simulink model "Observadores_Mimo"  (R2022b)
settings: Solver=ode23t  StartTime=0.0  StopTime=5  MaxStep=1e-3  RelTol=1e-3
values from neighbouring files (symbols this model uses):
  Ac = reg.a    [Observdores_funcion_lqg.m]    (also in Observdores_pto_equilibrio.m)
  Ac_1 = [AL-BL*Kest-L*CL+L*DL*Kest, BL*Ki - L*DL*Ki ... (first row only)    [Observdores.m]
  Ac_2 = reg.a    [Observdores.m]    (also in Observdores_funcion_lqg.m; lqg_funcion.m)
  AL = double(subs(A,{a,b,c,d},{a1,b1,c1,d1}))    [Observdores.m]    (also in Observdores_funcion_lqg.m = double(subs(A,{x1,x2,x3,x4,u1,u2,u3,u4},{x10,x20,x30,x40,u10; Observdores_pto_equilibrio.m; Observdores_pto_equilibrio_discreto.m; Observdores_seguimiento_discreto.m)
  Bc = reg.b    [Observdores_funcion_lqg.m]    (also in Observdores_pto_equilibrio.m)
  Bc_1 = [-L ... (first row only)    [Observdores.m]
  Bc_2 = reg.b    [Observdores.m]    (also in Observdores_funcion_lqg.m; lqg_funcion.m)
  BL = double(subs(B,{a,b,c,d},{a1,b1,c1,d1}))    [Observdores.m]    (also in Observdores_funcion_lqg.m = double(subs(B,{x1,x2,x3,x4,u1,u2,u3,u4},{x10,x20,x30,x40,u10; Observdores_pto_equilibrio.m; Observdores_pto_equilibrio_discreto.m; Observdores_seguimiento_discreto.m)
  Cc = sys_d2.c    [Observdores.m]    (also in Observdores_funcion_lqg.m = reg.c; Observdores_pto_equilibrio.m = reg.c; Observdores_pto_equilibrio_discreto.m = -K)
  Cc_1 = [-Kest, Ki]    [Observdores.m]
  Cc_2 = reg.c    [Observdores.m]    (also in Observdores_funcion_lqg.m; lqg_funcion.m)
  Ccon = [-Kest Ki]    [Observdores_seguimiento_discreto.m]
  CL = [1 0 0 ... (first row only)    [Observdores.m]    (also in Observdores_funcion_lqg.m = [1 1 0 0; Observdores_pto_equilibrio.m; Observdores_pto_equilibrio_discreto.m; Observdores_seguimiento_discreto.m)
  Dc = reg.d    [Observdores_funcion_lqg.m]    (also in Observdores_pto_equilibrio.m; Observdores_pto_equilibrio_discreto.m = zeros(p,r))
  Dc_1 = zeros(p,r)    [Observdores.m]
  Dc_2 = reg.d    [Observdores.m]    (also in Observdores_funcion_lqg.m; lqg_funcion.m)
  Dcon = zeros(p,2*r)    [Observdores_seguimiento_discreto.m]
  DL = [0 0 0 ... (first row only)    [Observdores.m]    (also in Observdores_funcion_lqg.m = [0 0 0 0; Observdores_pto_equilibrio.m; Observdores_pto_equilibrio_discreto.m; Observdores_seguimiento_discreto.m)
  Gc = sys_d2.a    [Observdores.m]    (also in Observdores_pto_equilibrio.m = sys_c_dig.a; Observdores_pto_equilibrio_discreto.m = GL-HL*K-L*CL+L*DL*K)
  Gcon = [GL-HL*Kest-L*CL+L*DL*Kest, HL*Ki - L*DL*Ki ... (first row only)    [Observdores_seguimiento_discreto.m]
  GL = sysd.a    [Observdores_pto_equilibrio_discreto.m]    (also in Observdores_seguimiento_discreto.m)
  Hc = sys_c_dig.b    [Observdores_pto_equilibrio.m]    (also in Observdores_pto_equilibrio_discreto.m = L)
  Hcon = [zeros(n,r), L ... (first row only)    [Observdores_seguimiento_discreto.m]
  HL = sysd.b    [Observdores_pto_equilibrio_discreto.m]    (also in Observdores_seguimiento_discreto.m)
  K = place(Ahat,Bhat,delta)    [Observdores.m]
  Kest = K(:,1:n)    [Observdores.m]    (also in Observdores_seguimiento_discreto.m)
  Ki = -K(:,n+1:end)    [Observdores.m]    (also in Observdores_seguimiento_discreto.m)
  L = (place(AL',CL',delta))'    [Observdores.m]    (also in Observdores_pto_equilibrio.m; Observdores_pto_equilibrio_discreto.m = place(GL',CL',pol_obv_d)'; Observdores_seguimiento_discreto.m = place(GL',CL',pol_obv_d)')
  sys_d1 = c2d(sys_c1,Tm)    [Observdores.m]
  sys_d2 = c2d(sys_c2,Tm)    [Observdores.m]
  Tm = 0.02    [Observdores.m]    (also in Observdores_pto_equilibrio.m; Observdores_pto_equilibrio_discreto.m = 0.05; Observdores_seguimiento_discreto.m = 0.05)
  u10 = (a1*x20 + b1*x10^2)/u20    [Observdores.m]    (also in Observdores_funcion_lqg.m = 1; Observdores_pto_equilibrio.m; Observdores_pto_equilibrio_discreto.m; Observdores_seguimiento_discreto.m)
  u20 = sqrt(c1*x30*x20)    [Observdores.m]    (also in Observdores_funcion_lqg.m = sqrt(x30*x20); Observdores_pto_equilibrio.m; Observdores_pto_equilibrio_discreto.m; Observdores_seguimiento_discreto.m)
  u30 = (d1*x30 - u10)/x10    [Observdores.m]    (also in Observdores_funcion_lqg.m = (x20 + x10^2 - u20^2)/u10; Observdores_pto_equilibrio.m; Observdores_pto_equilibrio_discreto.m; Observdores_seguimiento_discreto.m)
  x10 = 2    [Observdores.m]    (also in Observdores_funcion_lqg.m; Observdores_pto_equilibrio.m; Observdores_pto_equilibrio_discreto.m; Observdores_seguimiento_discreto.m)
  x20 = 4    [Observdores.m]    (also in Observdores_funcion_lqg.m = 8; Observdores_pto_equilibrio.m; Observdores_pto_equilibrio_discreto.m; Observdores_seguimiento_discreto.m)
  x30 = 4    [Observdores.m]    (also in Observdores_funcion_lqg.m = 2; Observdores_pto_equilibrio.m; Observdores_pto_equilibrio_discreto.m; Observdores_seguimiento_discreto.m)
  xini = [0.5; -0.3; -0.7; 0.9]    [Observdores_funcion_lqg.m]    (also in Observdores_pto_equilibrio.m = [0.2; -0.3; -0.4]; Observdores_pto_equilibrio_discreto.m = [0.2; -0.3; -0.4])
undefined symbols (not defined in the file or in its folder): magnitude
libraries: simulink x22
(part 3 of 3)

== matlab function Observadores_Mimo/Comparacion/MATLAB Function3 ==
  data: Sp input; ut output; Pv input; Con_in input; Con_out output
function [ut,Con_out] = fcn(Sp,Pv,Con_in)
Vk_1 = Con_in(1:2); % Número de integradores
Xk_1 = Con_in(3:5); % Estados planta
Du = Con_in(6:8); % Actuadores

u1max = 10;
u1min = -10;
u2max = 10;
u2min = -10;
u3max = 10;
u3min = -10;
u4max = 10;
u4min = -10;
Ka = zeros(2,3);  %(r,p)

GL = [0.449639072151396	-0.0615751578519137	0.00688879884775241
-0.0103331982716286	0.819090019262878	-0.167927508214218
0.0949460363457777	-0.00516659913581431	0.861071896316432];
HL = [0.137811004816424	0.191992740153676	0.000252311833454837
-0.00521058225806007	0.361441493724063	-0.00890729351539111
0.0575256575832432	0.0158782651576252	0.0928710476225001];
CL = [1	0	0
0	0	1];
Ki = [0.495926463268089	0.0790916425769034
0.300095646296171	0.0155567242100712
-0.211852960593149	0.275825414863402];
Kest = [0.507477329350552	-0.352045881677806	0.562420881396554
0.247771497752502	0.347060818569204	-0.103614364293038
0.0518961155196881	0.0183168185614278	1.23984083631819];
L = [0.0236567937142856	0.00882380149521764
0.0520705602169565	-0.0103631100189368
0.0214783272972567	0.0442958071558840];

en = Sp-Pv;
Vk = en + Vk_1 - Ka*Du;
u = Ki*Vk - Kest*Xk_1;
Xob = (GL-L*CL)*Xk_1 + HL*u + L*Pv;

u1s = u(1);
u2s = u(2);
u3s = u(3);

if u(1)>=u1max
    u1s = u1max;
end
if u(1)<=u1min
    u1s = u1min;
end

if u(2)>=u2max
    u2s = u2max;
end
if u(2)<=u2min
    u2s = u2min;
end

if u(3)>=u3max
    u3s = u3max;
end
if u(3)<=u3min
    u3s = u3min;
end

%% Salida
ut = [u1s;u2s;u3s];
Dunew = u - ut;
Con_out = [Vk; Xob; Dunew];

== matlab function Observadores_Mimo/Comparacion/Subsystem6/MATLAB Function ==
  data: x input; f output; u1 input; u2 input; u3 input
function f = fcn(x,u1,u2,u3)

x1 = x(1);
x2 = x(2);
x3 = x(3);

a = 2;
b = 4;
c = 1;
d = 3;

f1 = -a*x2 - b*x1^2 + u1*u2;
f2 = -c*x3*x2 + u2^2 ;
f3 = -d*x3 + u3*x1 + u1;

f = [f1;f2;f3];

== matlab function Observadores_Mimo/Control Estados_1 DOF_Unificado/MATLAB Function2 ==
  data: Sp input; ut output; Pv input; Con_ini input; Con_out output
function [ut,Con_out] = fcn(Sp,Pv,Con_ini)
Gc = [0.939974592711359	-2.37159326323049e-12	-0.00286835310590601	0.0698167323415246	-0.00133465785652806
-0.000328954995677950	0.802518797962479	0.00531052595531562	-1.22918191880968e-05	0.00254152882572689
-0.00286835310583805	4.00834161597228e-15	0.759858388826903	-0.000109199276806931	0.769506721453615
0	0	0	1	0
0	0	0	0	1];
Hc = [-0.00537081940417820	-0.00326725714133668
-0.000338557035146039	0.00607025843071000
-0.00295366005744958	-0.00876393614924446
0.0100000000000000	0
0	0.0100000000000000];
Cc = [2.60000000006463	3.87499999993181	-0.750000000024670	1.79999999984347	9.96447369061571e-11
-4.30872282297656e-11	-2.25000000000000	0.499999999999999	1.04354552776798e-10	1.64313007644523e-14
-2.80000000007810	-1.93749999996589	-11.1249999999877	-0.899999999768644	43.9999999999502];
Dc = [0	0
0	0
0	0];

u1max = 10;
u1min = -10;
u2max = 10;
u2min = -10;
u3max = 10;
u3min = -10;

Ka = zeros(5,3);  % (n+r,p)

xk = Con_ini(1:5);  %n+r
Du = Con_ini(6:8);  %p

error = Sp-Pv;
u = Cc*xk + Dc*error;
xk_1 = Gc*xk + Hc*error - Ka*Du;

u1s = u(1);
u2s = u(2);
u3s = u(3);

if u(1)>=u1max
    u1s = u1max;
end
if u(1)<=u1min
    u1s = u1min;
end

if u(2)>=u2max
    u2s = u2max;
end
if u(2)<=u2min
    u2s = u2min;
end

if u(3)>=u3max
    u3s = u3max;
end
if u(3)<=u3min
    u3s = u3min;
end

%% Salida
ut = [u1s;u2s;u3s];
Dunew = u - ut;
Con_out = [xk_1; Dunew];

== matlab function Observadores_Mimo/Control Estados_Punto Equilibrio_Discret_Codigo/MATLAB Function ==
  data: Pv input; ut output; Con_ini input; Con_out output
function [ut,Con_out] = fcn(Pv,Con_ini)
Gc = [0.423094793522468	-0.0746380079945671	7.31048780287791e-06
-0.0636860426356503	0.790816757730642	-0.142538588641518
0.0716883663040384	-0.00432635287691224	0.810485721297092];
Hc = [0.0236567937142856	0.00882380149521764
0.0520705602169565	-0.0103631100189368
0.0214783272972567	0.0442958071558840];
Cc = [-0.0153774129846732	0.0134134061965922	-0.0412224049065605
-0.00398999177371588	-0.0776847225572359	0.0397701338324362
-0.00895212043509818	0.0140208375355596	-0.0489980759438155];
Dc = [0	0
0	0
0	0];

u1max = 10;
u1min = -10;
u2max = 10;
u2min = -10;
u3max = 10;
u3min = -10;

xk = Con_ini;
u = Cc*xk + Dc*Pv;
xk_1 = Gc*xk + Hc*Pv;

u1s = u(1);
u2s = u(2);
u3s = u(3);

if u(1)>=u1max
    u1s = u1max;
end
if u(1)<=u1min
    u1s = u1min;
end

if u(2)>=u2max
    u2s = u2max;
end
if u(2)<=u2min
    u2s = u2min;
end

if u(3)>=u3max
    u3s = u3max;
end
if u(3)<=u3min
    u3s = u3min;
end

%% Salida
ut = [u1s;u2s;u3s];
Con_out = xk_1;

== matlab function Observadores_Mimo/Control Estados_Punto Equilibrio/Subsystem2/MATLAB Function ==
  data: x input; f output; u1 input; u2 input; u3 input
function f = fcn(x,u1,u2,u3)

x1 = x(1);
x2 = x(2);
x3 = x(3);

a = 2;
b = 4;
c = 1;
d = 3;

f1 = -a*x2 - b*x1^2 + u1*u2;
f2 = -c*x3*x2 + u2^2 ;
f3 = -d*x3 + u3*x1 + u1;

f = [f1;f2;f3];

== matlab function Observadores_Mimo/Control Estados_Punto Equilibrio_Unificado/MATLAB Function1 ==
  data: Pv input; ut output; Con_ini input; Con_out output
function [ut,Con_out] = fcn(Pv,Con_ini)
Gc = [0.639675637348658	-0.0775455511538108	-0.0361775651328436
-0.0279786075427977	0.839840756016632	-0.0327212601781411
0.00858159444938535	0.00353264359638387	0.876128273931381];
Hc = [0.0799079091258568	0.0343958926319344
0.0152867884447592	-0.0198265632532611
0.0407058310137895	0.0487236812197195];
Cc = [-0.168078279179797	0.0841565809088256	-0.289679004961983
-0.116738169404316	-0.601785811526129	0.131735649809089
-0.0556574417700977	0.0746769937798451	-0.356728242843576];
Dc = [0	0
0	0
0	0];

u1max = 10;
u1min = -10;
u2max = 10;
u2min = -10;
u3max = 10;
u3min = -10;

xk = Con_ini;
u = Cc*xk + Dc*Pv;
xk_1 = Gc*xk + Hc*Pv;

u1s = u(1);
u2s = u(2);
u3s = u(3);

if u(1)>=u1max
    u1s = u1max;
end
if u(1)<=u1min
    u1s = u1min;
end

if u(2)>=u2max
    u2s = u2max;
end
if u(2)<=u2min
    u2s = u2min;
end

if u(3)>=u3max
    u3s = u3max;
end
if u(3)<=u3min
    u3s = u3min;
end


%% Salida
ut = [u1s;u2s;u3s];
Con_out = xk_1;

== matlab function Observadores_Mimo/Control Estados_Discreto_2 DOF Unificado/Subsystem/MATLAB Function ==
  data: x input; f output; u1 input; u2 input; u3 input
function f = fcn(x,u1,u2,u3)

x1 = x(1);
x2 = x(2);
x3 = x(3);

a = 2;
b = 4;
c = 1;
d = 3;

f1 = -a*x2 - b*x1^2 + u1*u2;
f2 = -c*x3*x2 + u2^2 ;
f3 = -d*x3 + u3*x1 + u1;

f = [f1;f2;f3];

== matlab function Observadores_Mimo/Control Estados_Discreto_Codigo/Subsystem2/MATLAB Function ==
  data: x input; f output; u1 input; u2 input; u3 input
function f = fcn(x,u1,u2,u3)

x1 = x(1);
x2 = x(2);
x3 = x(3);

a = 2;
b = 4;
c = 1;
d = 3;

f1 = -a*x2 - b*x1^2 + u1*u2;
f2 = -c*x3*x2 + u2^2 ;
f3 = -d*x3 + u3*x1 + u1;

f = [f1;f2;f3];

== matlab function Observadores_Mimo/Control Estados_Punto Equilibrio_Discret_Codigo/MATLAB Function3 ==
  data: ut output; Pv input; Con_in input; Con_out output
function [ut,Con_out] = fcn(Pv,Con_in)
Xk_1 = Con_in; % Estados planta

u1max = 10;
u1min = -10;
u2max = 10;
u2min = -10;
u3max = 10;
u3min = -10;
Ka = zeros(2,4);  %(r,p)

GL = [0.449639072151396	-0.0615751578519137	0.00688879884775241
-0.0103331982716286	0.819090019262878	-0.167927508214218
0.0949460363457777	-0.00516659913581431	0.861071896316432];
HL = [0.137811004816424	0.191992740153676	0.000252311833454837
-0.00521058225806007	0.361441493724063	-0.00890729351539111
0.0575256575832432	0.0158782651576252	0.0928710476225001];
CL = [1	0	0
0	0	1];
DL = [0	0	0
0	0	0];
K = [0.0153774129846732	-0.0134134061965922	0.0412224049065605
0.00398999177371588	0.0776847225572359	-0.0397701338324362
0.00895212043509818	-0.0140208375355596	0.0489980759438155];
L = [0.0236567937142856	0.00882380149521764
0.0520705602169565	-0.0103631100189368
0.0214783272972567	0.0442958071558840];

u = -K*Xk_1;
Xob = GL*Xk_1 + HL*u + L*(Pv - CL*Xk_1 - DL*u);

u1s = u(1);
u2s = u(2);
u3s = u(3);

if u(1)>=u1max
    u1s = u1max;
end
if u(1)<=u1min
    u1s = u1min;
end

if u(2)>=u2max
    u2s = u2max;
end
if u(2)<=u2min
    u2s = u2min;
end

if u(3)>=u3max
    u3s = u3max;
end
if u(3)<=u3min
    u3s = u3min;
end


%% Salida
ut = [u1s;u2s;u3s];
Con_out = Xob;

== matlab function Observadores_Mimo/Control Estados_Discreto_Codigo/MATLAB Function1 ==
  data: Sp input; ut output; Pv input; Con_in input; Con_out output
function [ut,Con_out] = fcn(Sp,Pv,Con_in)
Vk_1 = Con_in(1:2); % Número de integradores
Xk_1 = Con_in(3:5); % Estados planta
Du = Con_in(6:8); % Actuadores

u1max = 10;
u1min = -10;
u2max = 10;
u2min = -10;
u3max = 10;
u3min = -10;
u4max = 10;
u4min = -10;
Ka = zeros(2,3);  %(r,p)

GL = [0.449639072151396	-0.0615751578519137	0.00688879884775241
-0.0103331982716286	0.819090019262878	-0.167927508214218
0.0949460363457777	-0.00516659913581431	0.861071896316432];
HL = [0.137811004816424	0.191992740153676	0.000252311833454837
-0.00521058225806007	0.361441493724063	-0.00890729351539111
0.0575256575832432	0.0158782651576252	0.0928710476225001];
CL = [1	0	0
0	0	1];
Ki = [0.495926463268089	0.0790916425769034
0.300095646296171	0.0155567242100712
-0.211852960593149	0.275825414863402];
Kest = [0.507477329350552	-0.352045881677806	0.562420881396554
0.247771497752502	0.347060818569204	-0.103614364293038
0.0518961155196881	0.0183168185614278	1.23984083631819];
L = [0.0236567937142856	0.00882380149521764
0.0520705602169565	-0.0103631100189368
0.0214783272972567	0.0442958071558840];

en = Sp-Pv;
Vk = en + Vk_1 - Ka*Du;
u = Ki*Vk - Kest*Xk_1;
Xob = (GL-L*CL)*Xk_1 + HL*u + L*Pv;

u1s = u(1);
u2s = u(2);
u3s = u(3);

if u(1)>=u1max
    u1s = u1max;
end
if u(1)<=u1min
    u1s = u1min;
end

if u(2)>=u2max
    u2s = u2max;
end
if u(2)<=u2min
    u2s = u2min;
end

if u(3)>=u3max
    u3s = u3max;
end
if u(3)<=u3min
    u3s = u3min;
end

%% Salida
ut = [u1s;u2s;u3s];
Dunew = u - ut;
Con_out = [Vk; Xob; Dunew];

== matlab function Observadores_Mimo/Control Estados_2 DOF_Unificado/MATLAB Function2 ==
  data: Sp input; u output; Pv input; Con_ini input; Con_out output
function [u,Con_out] = fcn(Sp,Pv,Con_ini)
Gc = [0.883560462392427	-4.13249708388486e-12	-0.00487572121212935	0.135443000110772	-0.00479641932613010
-0.000588434369415533	0.644036421083143	0.00829798816152157	-4.57027036271401e-05	0.00866807794337489
-0.00487572121200123	1.30651084000254e-14	0.577392998520158	-0.000392434304393785	1.35422668727884
0	0	0	1	0
0	0	0	0	1];
Hc = [0.00138236824312267	-3.37592528540001e-05	0.00971261372273124	0.00632660435715394
-3.16147125121532e-07	6.26926980241918e-05	0.000624297068749436	-0.0109217038882698
-2.76212064284266e-06	0.0147757234577708	0.00518371001609480	0.00771884768968612
0.0200000000000000	0	-0.0200000000000000	0
0	0.0200000000000000	0	-0.0200000000000000];
Cc = [2.60000000006463	3.87499999993181	-0.750000000024670	1.79999999984347	9.96447369061571e-11
-4.30872282297656e-11	-2.25000000000000	0.499999999999999	1.04354552776798e-10	1.64313007644523e-14
-2.80000000007810	-1.93749999996589	-11.1249999999877	-0.899999999768644	43.9999999999502];
Dc = [0	0	0	0
0	0	0	0
0	0	0	0];

u1max = 10;
u1min = -10;
u2max = 10;
u2min = -10;
u3max = 10;
u3min = -10;

Ka = zeros(5,3);

xk = Con_ini(1:5);  %n+r
Du = Con_ini(6:8);  %p

u = Cc*xk + Dc*[Sp;Pv];
xk_1 = Gc*xk + Hc*[Sp;Pv] - Ka*Du;

% Hsp = [0.000536712016934462,0.000277774040110453;0.00110188262899529,-0.000214997449972678;5.70600160926339e-05,0.000178431372314633;0.000111261745162715,-0.000748573895925450;0.0600000000000000,0;0,0.0600000000000000];
% Hpv = [0.528743127428489,-0.0440381830752178;0.441160175174069,0.0425524022491926;-0.00772595368821204,0.204727393044363;-0.0185719938075179,0.0357506408044768;-0.0600000000000000,0;0,-0.0600000000000000];
% u = Cc*xk;
% xk_1 = Gc*xk + Hsp*Sp + Hpv*Pv - Ka*Du;

u1s = u(1);
u2s = u(2);
u3s = u(3);

if u(1)>=u1max
    u1s = u1max;
end
if u(1)<=u1min
    u1s = u1min;
end

if u(2)>=u2max
    u2s = u2max;
end
if u(2)<=u2min
    u2s = u2min;
end

if u(3)>=u3max
    u3s = u3max;
end
if u(3)<=u3min
    u3s = u3min;
end

%% Salida
ut = [u1s;u2s;u3s];
Dunew = u - ut;
Con_out = [xk_1; Dunew];

== matlab function Observadores_Mimo/Control Estados_2 DOF_Unificado/MATLAB Function1 ==
  data: Sp input; u output; Pv input; Con_ini input; Con_out output
function [u,Con_out] = fcn(Sp,Pv,Con_ini)
Gc = [0.883560462392427	-4.13249708388486e-12	-0.00487572121212935	0.135443000110772	-0.00479641932613010
-0.000588434369415533	0.644036421083143	0.00829798816152157	-4.57027036271401e-05	0.00866807794337489
-0.00487572121200123	1.30651084000254e-14	0.577392998520158	-0.000392434304393785	1.35422668727884
0	0	0	1	0
0	0	0	0	1];
Hc = [0.00138236824312267	-3.37592528540001e-05	0.00971261372273124	0.00632660435715394
-3.16147125121532e-07	6.26926980241918e-05	0.000624297068749436	-0.0109217038882698
-2.76212064284266e-06	0.0147757234577708	0.00518371001609480	0.00771884768968612
0.0200000000000000	0	-0.0200000000000000	0
0	0.0200000000000000	0	-0.0200000000000000];
Cc = [2.60000000006463	3.87499999993181	-0.750000000024670	1.79999999984347	9.96447369061571e-11
-4.30872282297656e-11	-2.25000000000000	0.499999999999999	1.04354552776798e-10	1.64313007644523e-14
-2.80000000007810	-1.93749999996589	-11.1249999999877	-0.899999999768644	43.9999999999502];
Dc = [0	0	0	0
0	0	0	0
0	0	0	0];

u1max = 10;
u1min = -10;
u2max = 10;
u2min = -10;
u3max = 10;
u3min = -10;

Ka = zeros(5,3);

xk = Con_ini(1:5);  %n+r
Du = Con_ini(6:8);  %p

u = Cc*xk + Dc*[Sp;Pv];
xk_1 = Gc*xk + Hc*[Sp;Pv] - Ka*Du;

% Hsp = [0.000536712016934462,0.000277774040110453;0.00110188262899529,-0.000214997449972678;5.70600160926339e-05,0.000178431372314633;0.000111261745162715,-0.000748573895925450;0.0600000000000000,0;0,0.0600000000000000];
% Hpv = [0.528743127428489,-0.0440381830752178;0.441160175174069,0.0425524022491926;-0.00772595368821204,0.204727393044363;-0.0185719938075179,0.0357506408044768;-0.0600000000000000,0;0,-0.0600000000000000];
% u = Cc*xk;
% xk_1 = Gc*xk + Hsp*Sp + Hpv*Pv - Ka*Du;

u1s = u(1);
u2s = u(2);
u3s = u(3);

if u(1)>=u1max
    u1s = u1max;
end
if u(1)<=u1min
    u1s = u1min;
end

if u(2)>=u2max
    u2s = u2max;
end
if u(2)<=u2min
    u2s = u2min;
end

if u(3)>=u3max
    u3s = u3max;
end
if u(3)<=u3min
    u3s = u3min;
end

%% Salida
ut = [u1s;u2s;u3s];
Dunew = u - ut;
Con_out = [xk_1; Dunew];

== matlab function Observadores_Mimo/Control Estados_Punto Equilibrio_Unificado/MATLAB Function2 ==
  data: Pv input; ut output; Con_ini input; Con_out output
function [ut,Con_out] = fcn(Pv,Con_ini)
Gc = [0.639675637348658	-0.0775455511538108	-0.0361775651328436
-0.0279786075427977	0.839840756016632	-0.0327212601781411
0.00858159444938535	0.00353264359638387	0.876128273931381];
Hc = [0.0799079091258568	0.0343958926319344
0.0152867884447592	-0.0198265632532611
0.0407058310137895	0.0487236812197195];
Cc = [-0.168078279179797	0.0841565809088256	-0.289679004961983
-0.116738169404316	-0.601785811526129	0.131735649809089
-0.0556574417700977	0.0746769937798451	-0.356728242843576];
Dc = [0	0
0	0
0	0];

u1max = 10;
u1min = -10;
u2max = 10;
u2min = -10;
u3max = 10;
u3min = -10;

xk = Con_ini;
u = Cc*xk + Dc*Pv;
xk_1 = Gc*xk + Hc*Pv;

u1s = u(1);
u2s = u(2);
u3s = u(3);

if u(1)>=u1max
    u1s = u1max;
end
if u(1)<=u1min
    u1s = u1min;
end

if u(2)>=u2max
    u2s = u2max;
end
if u(2)<=u2min
    u2s = u2min;
end

if u(3)>=u3max
    u3s = u3max;
end
if u(3)<=u3min
    u3s = u3min;
end


%% Salida
ut = [u1s;u2s;u3s];
Con_out = xk_1;

== matlab function Observadores_Mimo/Comparacion/MATLAB Function1 ==
  data: Sp input; ut output; Pv input; Con_ini input; Con_out output
function [ut,Con_out] = fcn(Sp,Pv,Con_ini)
Gc = [0.939974592711359	-2.37159326323049e-12	-0.00286835310590601	0.0698167323415246	-0.00133465785652806
-0.000328954995677950	0.802518797962479	0.00531052595531562	-1.22918191880968e-05	0.00254152882572689
-0.00286835310583805	4.00834161597228e-15	0.759858388826903	-0.000109199276806931	0.769506721453615
0	0	0	1	0
0	0	0	0	1];
Hc = [-0.00537081940417820	-0.00326725714133668
-0.000338557035146039	0.00607025843071000
-0.00295366005744958	-0.00876393614924446
0.0100000000000000	0
0	0.0100000000000000];
Cc = [2.60000000006463	3.87499999993181	-0.750000000024670	1.79999999984347	9.96447369061571e-11
-4.30872282297656e-11	-2.25000000000000	0.499999999999999	1.04354552776798e-10	1.64313007644523e-14
-2.80000000007810	-1.93749999996589	-11.1249999999877	-0.899999999768644	43.9999999999502];
Dc = [0	0
0	0
0	0];

u1max = 10;
u1min = -10;
u2max = 10;
u2min = -10;
u3max = 10;
u3min = -10;

Ka = zeros(5,3);  % (n+r,p)

xk = Con_ini(1:5);  %n+r
Du = Con_ini(6:8);  %p

error = Sp-Pv;
u = Cc*xk + Dc*error;
xk_1 = Gc*xk + Hc*error - Ka*Du;

u1s = u(1);
u2s = u(2);
u3s = u(3);

if u(1)>=u1max
    u1s = u1max;
end
if u(1)<=u1min
    u1s = u1min;
end

if u(2)>=u2max
    u2s = u2max;
end
if u(2)<=u2min
    u2s = u2min;
end

if u(3)>=u3max
    u3s = u3max;
end
if u(3)<=u3min
    u3s = u3min;
end

%% Salida
ut = [u1s;u2s;u3s];
Dunew = u - ut;
Con_out = [xk_1; Dunew];

== matlab function Observadores_Mimo/Control Estados_Punto Equilibrio_Discreto/Subsystem2/MATLAB Function ==
  data: x input; f output; u1 input; u2 input; u3 input
function f = fcn(x,u1,u2,u3)

x1 = x(1);
x2 = x(2);
x3 = x(3);

a = 2;
b = 4;
c = 1;
d = 3;

f1 = -a*x2 - b*x1^2 + u1*u2;
f2 = -c*x3*x2 + u2^2 ;
f3 = -d*x3 + u3*x1 + u1;

f = [f1;f2;f3];

== matlab function Observadores_Mimo/Control Estados_Desacoplado/Subsystem/MATLAB Function ==
  data: x input; f output; u1 input; u2 input; u3 input
function f = fcn(x,u1,u2,u3)

x1 = x(1);
x2 = x(2);
x3 = x(3);

a = 2;
b = 4;
c = 1;
d = 3;

f1 = -a*x2 - b*x1^2 + u1*u2;
f2 = -c*x3*x2 + u2^2 ;
f3 = -d*x3 + u3*x1 + u1;

f = [f1;f2;f3];

== matlab function Observadores_Mimo/Control Estados_1 DOF_Unificado/Subsystem/MATLAB Function ==
  data: x input; f output; u1 input; u2 input; u3 input
function f = fcn(x,u1,u2,u3)

x1 = x(1);
x2 = x(2);
x3 = x(3);

a = 2;
b = 4;
c = 1;
d = 3;

f1 = -a*x2 - b*x1^2 + u1*u2;
f2 = -c*x3*x2 + u2^2 ;
f3 = -d*x3 + u3*x1 + u1;

f = [f1;f2;f3];
